simulink subsystem "missile"  (R2024a)
settings: Solver=VariableStepAuto  StartTime=0.0  StopTime=10.0  RelTol=1e-3
values from neighbouring files (symbols this model uses):
  A = [-1.064 1.000; 290.26 0.00]    [Effect_of_Q.m]    (also in LQR.m; LQR_PI.m; PD_drd.m = [-0.0089  -0.1474     0   -9.75; Pure_LQR.m = [-1.064   1.000)
  B = [-0.25; -331.40]    [Effect_of_Q.m]    (also in LQR.m; LQR_PI.m; PD_drd.m = [0; Pure_LQR.m = [-0.25)
  C = [-123.34 0.00; 0.00 1.00]    [Effect_of_Q.m]    (also in LQR.m; LQR_PI.m; PD_drd.m = eye(4); Pure_LQR.m = [-123.34   0.00)
  D = [0; 0]    [Effect_of_Q.m]    (also in LQR.m; LQR_PI.m; PD_drd.m = zeros(4,1); Pure_LQR.m = [-13.51)
  dt1 = 0.75    [main.m]
  dt2 = 0.25    [main.m]
  K = dlqr(Ad, Bd, Q, R)    [LQR.m]    (also in StateFeedbackController.m = K_aug(1:2); run_missile_controller.m = K_aug(1:2))
undefined symbols (not defined in the file or in its folder): L
libraries: simulink x2
settings Model: Creator=Siddarth  LastModifiedBy=Siddarth

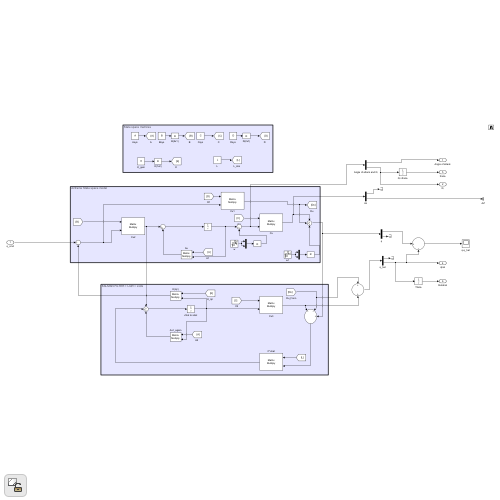
[thumbnail: Simulink's stored preview of the top-level diagram]
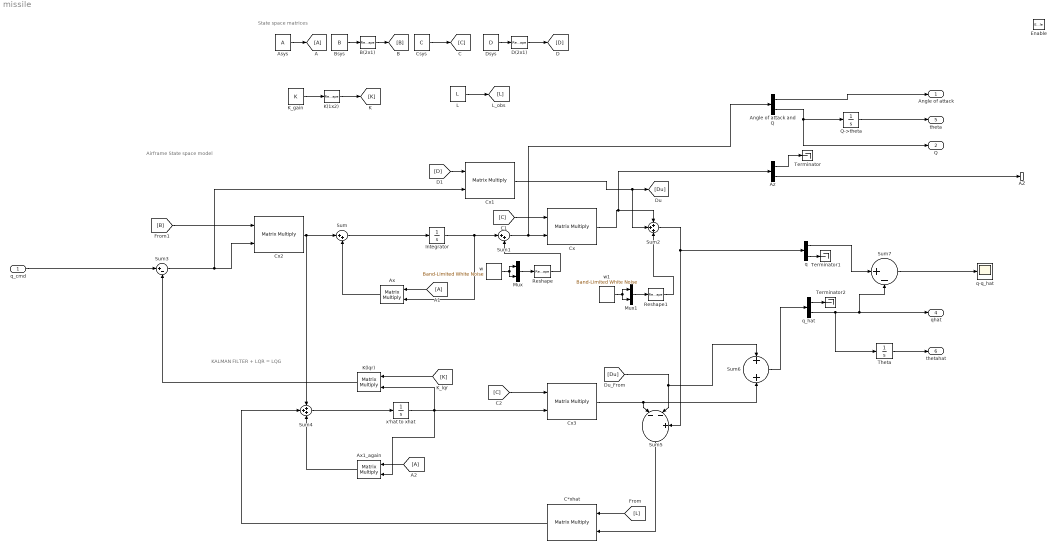
== system missile ==
  note: KALMAN FILTER + LQR = LQG
  note: Airframe State space model
  note: State space matrices
  q_cmd : Inport
  Enable : EnablePort
  A : Goto
  A1 : From
  A2 : From
  Angle of attack and Q : Demux  Outputs=2
  Asys : Constant  Value=A
  Ax : Product  Multiplication=Matrix(*)
  Ax1_again : Product  Multiplication=Matrix(*)
  Az : Demux  Outputs=2
  B(2x1) : Reshape  OutputDimensionality=Customize  OutputDimensions=[2,1]
  Bsys : Constant  Value=B
  C*xhat : Product  Multiplication=Matrix(*)
  Csys : Constant  Value=C
  Cx{,1..3} (4 alike) : Product  Multiplication=Matrix(*)
  D(2x1) : Reshape  OutputDimensionality=Customize  OutputDimensions=[2,1]
  Dsys : Constant  Value=D
  Integrator : Integrator
  K(1x2) : Reshape  OutputDimensionality=Customize  OutputDimensions=[1,2]
  K(lqr) : Product  Multiplication=Matrix(*)
  K_gain : Constant  Value=K
  L : Constant  Value=L
  Mux : Mux  Inputs=2
  Mux1 : Mux  Inputs=2
  Q->theta : Integrator
  Reshape : Reshape  OutputDimensionality=Customize  OutputDimensions=[2,1]
  Reshape1 : Reshape  OutputDimensionality=Customize  OutputDimensions=[2,1]
  Sum : Sum  Inputs=|++
  Sum1 : Sum  Inputs=|++
  Sum2 : Sum  Inputs=+++
  Sum3 : Sum  Inputs=|+-
  Sum4 : Sum  Inputs=+++
  Sum5 : Sum  Inputs=|--+
  Sum6 : Sum
  Sum7 : Sum  Inputs=|+-
  Terminator : Terminator
  Terminator1 : Terminator
  Terminator2 : Terminator
  Theta : Integrator
  q : Demux  Outputs=2
  q-q_hat : Scope
  q_hat : Demux  Outputs=2
  w : simulink/Sources/Band-Limited White Noise  Cov=[0.0000001]  Ts=dt1  seed=[23341]
  w1 : simulink/Sources/Band-Limited White Noise  Cov=[0.00001]  Ts=dt2  seed=[23341]
  x'hat to xhat : Integrator
  Angle of attack : Outport
  Q : Outport  Port=2
  AZ : Outport  Port=3
  qhat : Outport  Port=4
  theta : Outport  Port=5
  thetahat : Outport  Port=6
  wires:
  K(1x2)/1 -> [K]
  Sum2/1 -> Sum5/3, q/1
  q/2 -> Terminator1/1
  [K] -> K(lqr)/1
  Integrator/1 -> Sum1/1, Ax/2
  Csys/1 -> [C]
  Sum1/1 -> Cx/2, Angle of attack and Q/1
  Sum3/1 -> Cx2/2, Cx1/2
  [C] -> Cx/1
  K_gain/1 -> K(1x2)/1
  w1/1 -> Mux1/2, Mux1/1
  Angle of attack and Q/2 -> Q->theta/1, Q/1
  Sum7/1 -> q-q_hat/1
  Ax1_again/1 -> Sum4/3
  x'hat to xhat/1 -> Cx3/2, K(lqr)/2, Ax1_again/2
  Cx3/1 -> Sum5/1, Sum6/2
  Bsys/1 -> B(2x1)/1
  Theta/1 -> thetahat/1
  Asys/1 -> A/1
  [B] -> Cx2/1
  A1/1 -> Ax/1
  L/1 -> [L]
  q_hat/2 -> Sum7/2, qhat/1, Theta/1
  Az/2 -> AZ/1
  Sum4/1 -> x'hat to xhat/1
  Reshape/1 -> Sum1/2
  w/1 -> Mux/2, Mux/1
  K(lqr)/1 -> Sum3/2
  [C] -> Cx3/1
  Ax/1 -> Sum/2
  Cx1/1 -> Sum2/2, [Du]
  Az/1 -> Terminator/1
  Cx2/1 -> Sum4/1, Sum/1
  C*xhat/1 -> Sum4/2
  A2/1 -> Ax1_again/1
  [Du] -> Sum5/2, Sum6/1
  Sum/1 -> Integrator/1
  Sum5/1 -> C*xhat/2
  Reshape1/1 -> Sum2/3
  Cx/1 -> Sum2/1, Az/1
  q_hat/1 -> Terminator2/1
  [D] -> Cx1/1
  Mux/1 -> Reshape/1
  Sum6/1 -> q_hat/1
  Mux1/1 -> Reshape1/1
  [L] -> C*xhat/1
  q/1 -> Sum7/1
  Q->theta/1 -> theta/1
  Angle of attack and Q/1 -> Angle of attack/1
  B(2x1)/1 -> [B]
  q_cmd/1 -> Sum3/1
  D(2x1)/1 -> [D]
  Dsys/1 -> D(2x1)/1
